simulink model "Subsystem"  (R2016a)
settings: Solver=VariableStepAuto  StartTime=0.0  StopTime=0.5  RelTol=1e-3
libraries: simulink x2, powerlib_meascontrol x1
settings Model: Creator=syf  LastModifiedBy=syf
settings DataIOCC: SaveOutput=off  SaveTime=off
settings DebuggingCC: AlgebraicLoopMsg=none

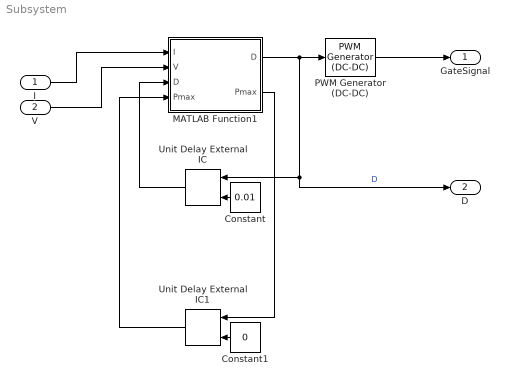
== system Subsystem ==
  I : Inport  OutDataTypeStr=double  PortDimensions=1  SampleTime=0
  V : Inport  Port=2  OutDataTypeStr=double  PortDimensions=1  SampleTime=0
  Constant : Constant  Value=0.01
  Constant1 : Constant  Value=0
  MATLAB Function1 : MATLAB Function  TreatAsAtomicUnit=on
  PWM Generator (DC-DC) : powerlib_meascontrol/Pulse & Signal Generators/PWM Generator (DC-DC)  Fsw=20000  Ts=0
  Unit Delay External IC : simulink/Additional Math & Discrete/Additional Discrete/Unit Delay External IC  tsamp=0.1
  Unit Delay External IC1 : simulink/Additional Math & Discrete/Additional Discrete/Unit Delay External IC  tsamp=0.1
  GateSignal : Outport  OutDataTypeStr=double  PortDimensions=1  SampleTime=[0,1]
  D : Outport  Port=2  OutDataTypeStr=double  PortDimensions=1  SampleTime=0
  wires:
  Unit Delay External IC1/1 -> MATLAB Function1/4("Pmax ")
  MATLAB Function1/2(Pmax) -> Unit Delay External IC1/1
  Unit Delay External IC/1 -> MATLAB Function1/3("D ")
  PWM Generator (DC-DC)/1 -> GateSignal/1
  Constant/1 -> Unit Delay External IC/2
  Constant1/1 -> Unit Delay External IC1/2
  I/1 -> MATLAB Function1/1(I)
  V/1 -> MATLAB Function1/2(V)
  MATLAB Function1/1(D) -> Unit Delay External IC/1, D/1, PWM Generator (DC-DC)/1  "D"

== matlab function Subsystem/MATLAB Function1 ==
  data: I input; D output; V input; D input; Pmax input; Pmax output
function [D, Pmax] = fcn(I,V,D,Pmax)
    P=I*V;
    if (D<1) && (D>0)
        if (P>Pmax) 
        D=D+0.01;
        Pmax=P;
        end
         if (P<Pmax)
            D=D-0.01;
         end
         if(P==Pmax)
            Pmax=P;
         end
    end
